simulink model "blockPID"  (R2017a)
settings: Solver=VariableStepAuto  StartTime=0.0  StopTime=1  RelTol=1e-3
values from neighbouring files (symbols this model uses):
  C = k*(kp + kd*s)    [maglev_values.m]
  I0 = sqrt(m*g*X0^2/C)    [maglev_values.m]
  L = 0.483    [maglev_values.m]
  m = 0.068    [maglev_values.m]
  R = 28    [maglev_values.m]
  X0 = 0.01    [maglev_values.m]
libraries: simulink x2
settings Model: Creator=alakmazaheri  LastModifiedBy=alakmazaheri

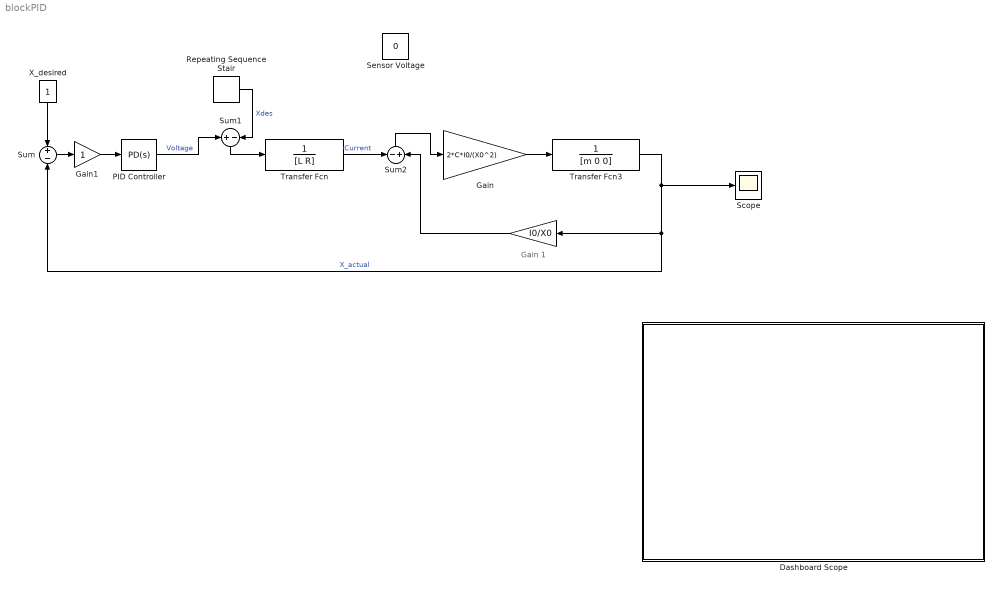
== system blockPID ==
  note: Gain 1
  " " : Gain  Gain=I0/X0
  Dashboard Scope : Subsystem  DialogController=hmiCreateDDGDialog  IsWebBlock=on  mask(MWDashboardBlock){webBlockId=e7fc13ea-75af-424b-a26f-d63fe7ac14b9, webBlockType=sdiscope, ShowInitialText=on, HMISrcModelName=blockPID}
      mask prompts: webBlockId "WebBlock Id"; webBlockType "WebBlock Type"; HMISrcModelName "Source Model"
      mask help: SimulinkHMI:dialogs:HMIScopeDialogDesc
      mask Help: helpview([docroot '/mapfiles/simulink.map'], 'hmi_scope')
      mask Display:
      | if strcmp(get_param(bdroot(gcb),'BlockDiagramType'), 'library')
      |     image([(matlabroot) '/toolbox/simulink/hmi/icons/DashboardScope.png']);
      | end
  Gain : Gain  Gain=2*C*I0/(X0^2)
  Gain1 : Gain
  PID Controller : simulink/Continuous/PID Controller  Controller=PD  TimeDomain=Continuous-time  SampleTime=-1  IntegratorMethod=Forward Euler  FilterMethod=Forward Euler  Form=Parallel  UseFilter=on  ControllerParametersSource=internal  P=30  I=0  D=1  N=100  InitialConditionSource=internal  InitialConditionForIntegrator=0  InitialConditionForFilter=0  ExternalReset=none  LimitOutput=off  UpperSaturationLimit=inf  LowerSaturationLimit=-inf  LinearizeAsGain=on  AntiWindupMode=none  Kb=1  TrackingMode=off  Kt=1  PParamMin=[]  PParamMax=[]  IParamMin=[]  IParamMax=[]  DParamMin=[]  DParamMax=[]  NParamMin=[]  NParamMax=[]  KbParamMin=[]  KbParamMax=[]  KtParamMin=[]  KtParamMax=[]  POutMin=[]  POutMax=[]  IOutMin=[]  IOutMax=[]  DOutMin=[]  DOutMax=[]  NOutMin=[]  NOutMax=[]  KbOutMin=[]  KbOutMax=[]  KtOutMin=[]  KtOutMax=[]  IntegratorOutMin=[]  IntegratorOutMax=[]  FilterOutMin=[]  FilterOutMax=[]  SumOutMin=[]  SumOutMax=[]  SumI1OutMin=[]  SumI1OutMax=[]  SumI2OutMin=[]  SumI2OutMax=[]  SumI3OutMin=[]  SumI3OutMax=[]  SumDOutMin=[]  SumDOutMax=[]  SaturationOutMin=[]  SaturationOutMax=[]  IntegratorContinuousStateAttributes=''  IntegratorStateMustResolveToSignalObject=off  IntegratorRTWStateStorageClass=Auto  FilterContinuousStateAttributes=''  FilterStateMustResolveToSignalObject=off  FilterRTWStateStorageClass=Auto  DifferentiatorICPrevScaledInput=0  DifferentiatorOutMin=[]  DifferentiatorOutMax=[]  InitialConditionSetting=State (most efficient)
  Repeating Sequence Stair : simulink/Sources/Repeating Sequence Stair  OutValues=[1 0]  tsamp=1  OutMin=[]  OutMax=[]  OutDataTypeStr=double  OutputDataTypeScalingMode=double  OutDataType=fixdt(0,8)  ConRadixGroup=Best Precision: Vector-wise  OutScaling=2^-12
  Scope : Scope
  Sensor Voltage : Constant  Value=0
  Sum : Sum  Inputs=+-
  Sum1 : Sum  Inputs=+-
  Sum2 : Sum  Inputs=-+
  Transfer Fcn : TransferFcn  Denominator=[L R]
  Transfer Fcn3 : TransferFcn  Denominator=[m 0 0]
  X_desired : Constant
  wires:
  Transfer Fcn/1 -> Sum2/1  "Current"
  Sum2/1 -> Gain/1
  Gain/1 -> Transfer Fcn3/1
  Transfer Fcn3/1 -> Scope/1, " "/1, Sum/2  "X_actual"
  Sum1/1 -> Transfer Fcn/1
  " "/1 -> Sum2/2
  X_desired/1 -> Sum/1
  Sum/1 -> Gain1/1
  PID Controller/1 -> Sum1/1  "Voltage"
  Gain1/1 -> PID Controller/1
  Repeating Sequence Stair/1 -> Sum1/2  "Xdes"

== system blockPID/Dashboard Scope ==
